simulink model "sb13_1d"  (Simulink 6.0)
settings: Solver=ode45  SolverMode=SingleTasking  StartTime=0.0  StopTime=999999  MaxStep=10  RelTol=1e-3  AbsTol=1e-6
values from neighbouring files (symbols this model uses):
  Gs = 10/(60*s+1)/(.1*s+1)    [m0108d.m]    (also in m0109b.m = 1/(8*s+1)^3; m0113c.m = 180/(.2*s+1)^3; m0251.m = b0/(a2*s^2+a1*s+a0); m0252.m = b0/(a2*s^2+a1*s+a0))
  Kpr = 10    [m0108d.m]    (also in m0109b.m = 1; m0113c.m; m0404Bsp.m = 3)
  sAdach = .2    (= 0.2)    [m0108d.m]    (also in m0113c.m)
  Tt = .4    (= 0.4)    [m0108d.m]    (also in m0259.m = 1; m0314.m = 2.13; m0322.m = 0.8; m0326.m = 4)
settings Model: LastModifiedBy=Froriep
settings DataIOCC: LimitDataPoints=off  SaveOutput=off  SaveTime=off
settings OptimizationCC: BooleanDataType=off
settings DebuggingCC: SolverPrmCheckMsg=none
settings HardwareCC: TargetUnknown=on

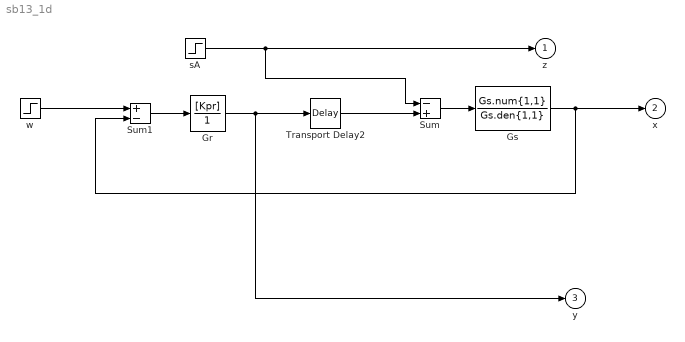
== system sb13_1d ==
  Gr : TransferFcn  Numerator=[Kpr]  Denominator=[1]
  Gs : TransferFcn  Numerator=Gs.num{1,1}  Denominator=Gs.den{1,1}
  Sum : Sum  Inputs=-+  SaturateOnIntegerOverflow=on  InputSameDT=on
  Sum1 : Sum  Inputs=+-  SaturateOnIntegerOverflow=on  InputSameDT=on
  Transport Delay2 : TransportDelay  DelayTime=Tt
  sA : Step  Time=.5  After=sAdach  SampleTime=0
  w : Step  After=0  SampleTime=0
  z : Outport  InitialOutput=0
  x : Outport  Port=2  InitialOutput=0
  y : Outport  Port=3  InitialOutput=0
  wires:
  Gr/1 -> y/1, Transport Delay2/1
  Sum1/1 -> Gr/1
  w/1 -> Sum1/1
  Gs/1 -> Sum1/2, x/1
  sA/1 -> z/1, Sum/1
  Sum/1 -> Gs/1
  Transport Delay2/1 -> Sum/2
